simulink model "NoThermalEffect"  (R2026b)
settings: Solver=VariableStepAuto
undefined symbols (not defined in the file): Qbatt, Qem, Qpwre
settings Model: ModifiedByFormat=The MathWorks, Inc.  Creator=The MathWorks, Inc.  LastModifiedBy=The MathWorks, Inc.

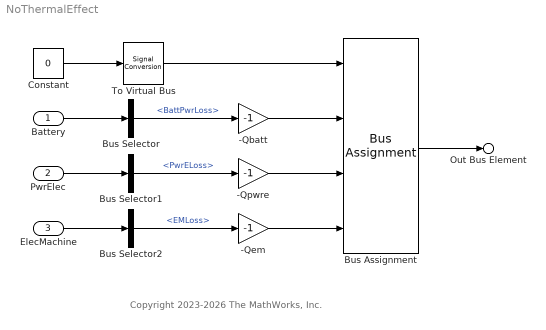
== system NoThermalEffect ==
  note: Copyright 2023-2026 The MathWorks, Inc.
  Battery : Inport
  PwrElec : Inport  Port=2
  ElecMachine : Inport  Port=3
  -Qbatt : Gain  Gain=-1
  -Qem : Gain  Gain=-1
  -Qpwre : Gain  Gain=-1
  Bus Assignment : BusAssignment  AssignedSignals=Qbatt,Qpwre,Qem
  Bus Selector : BusSelector  OutputSignals=BattInfo.BattPwrLoss
  Bus Selector1 : BusSelector  OutputSignals=PwrELoss
  Bus Selector2 : BusSelector  OutputSignals=EMPwrLoss  OutputAsBus=on
  Constant : Constant  Value=0  OutDataTypeStr=Bus: ThermalBUS  SampleTime=-1
  To Virtual Bus : SignalConversion  ConversionOutput=Virtual bus  OverrideOpt=off
  Out Bus Element : Outport  PortName=Thermal
  wires:
  Bus Assignment/1 -> Out Bus Element/1
  Bus Selector2/1 -> -Qem/1  "<EMLoss>"
  Bus Selector/1 -> -Qbatt/1  "<BattPwrLoss>"
  Battery/1 -> Bus Selector/1
  PwrElec/1 -> Bus Selector1/1
  Bus Selector1/1 -> -Qpwre/1  "<PwrELoss>"
  ElecMachine/1 -> Bus Selector2/1
  To Virtual Bus/1 -> Bus Assignment/1
  Constant/1 -> To Virtual Bus/1
  -Qpwre/1 -> Bus Assignment/3
  -Qem/1 -> Bus Assignment/4
  -Qbatt/1 -> Bus Assignment/2
